simulink model "drone_test-NOAHVUKOSA9F3D"  (R2021b)
settings: Solver=VariableStepAuto  StartTime=0.0  StopTime=10  RelTol=1e-3
values from neighbouring files (symbols this model uses):
  D = [Env.UnrealRiverPts(Env.RiverRegions(i,4),1) Env.UnrealRiverPts(Env.RiverRegions(i,4),2)]    [DefineUAVPath.m]    (also in DistributeIceXML.m; DistributeIceXML1.m; DroneSurveyRegions.m; EstimateIceNumerals.m)
libraries: uavsim3dlib x2, sim3dcameralib x1, sim3dphyssensorlib x1, sim3dlib x1, visionsinks x1
settings Model: Creator=zckog  LastModifiedBy=noahvukosa

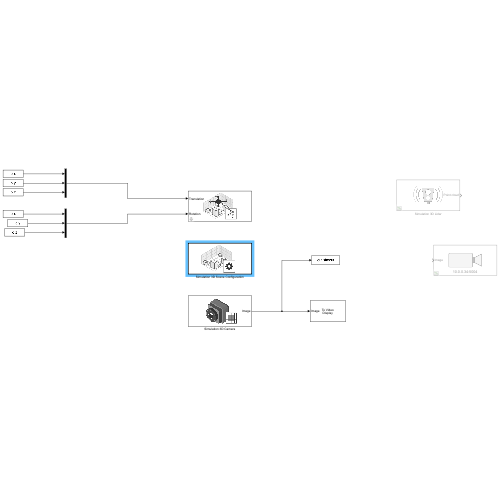
[thumbnail: Simulink's stored preview of the top-level diagram]
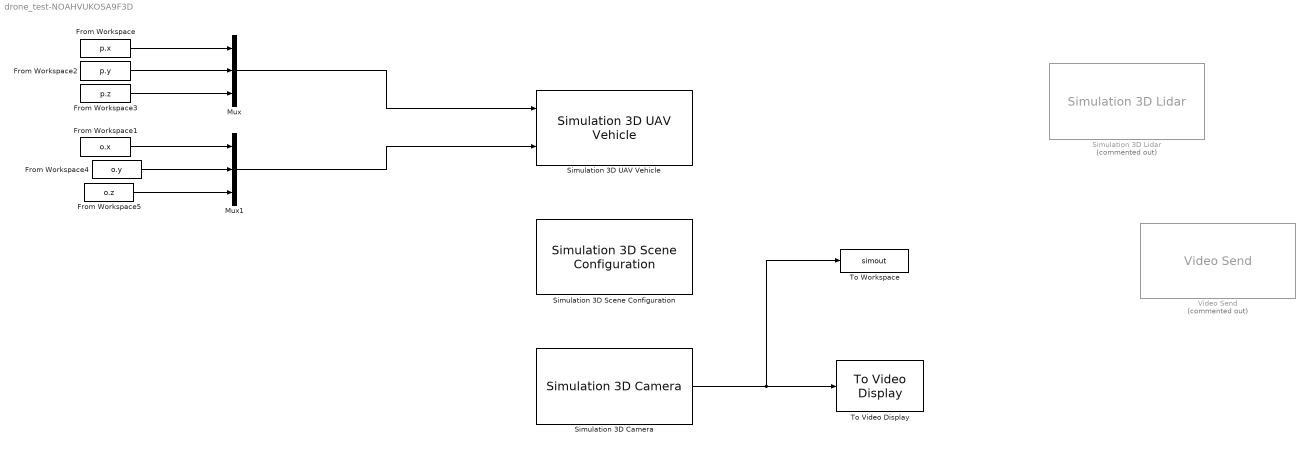
== system drone_test-NOAHVUKOSA9F3D ==
  From Workspace : FromWorkspace  VariableName=p.x
  From Workspace1 : FromWorkspace  VariableName=o.x
  From Workspace2 : FromWorkspace  VariableName=p.y
  From Workspace3 : FromWorkspace  VariableName=p.z
  From Workspace4 : FromWorkspace  VariableName=o.y
  From Workspace5 : FromWorkspace  VariableName=o.z
  Mux : Mux  Inputs=3
  Mux1 : Mux  Inputs=3
  Simulation 3D Camera : sim3dcameralib/Simulation 3D Camera  Priority=1  sensorTag=Sim3dSensor1  sensorId=1  sensorName=Sim3dSensor1  vehTagList={'Scene Origin';'SimulinkVehicle1'}  vehTag=SimulinkVehicle1  mountLoc=Origin  offsetFlag=on  tmountOffset=[0, 0, 0]  extTmount=off  rmountOffset=[0, pi/2, 0]  extRmount=off  FocalLength=[1109, 1109]  OpticalCenter=[640, 360]  ImageSize=[720, 1280]  RadialDistortion=[0, 0]  TangentialDistortion=[0, 0]  SensorSkew=0  DepthOutportEnabled=off  SemanticOutportEnabled=off  TransformOutportEnabled=off  SampleTime=-1  mountPoint=[0 0 0]  mountOrientation=[0 -1.5707963267949 0]  aMode=4  ID=1
      settings: SourceProductBaseCode=AE,DR,UV,VE
  Simulation 3D Lidar : sim3dphyssensorlib/Simulation 3D Lidar  Priority=1  Commented=on  sensorTag=Sim3dSensor2  sensorId=2  sensorName=Sim3dSensor2  vehTagList={'Scene Origin';'SimulinkVehicle1'}  vehTag=SimulinkVehicle1  mountLoc=Origin  offsetFlag=on  tmountOffset=[0, 0, 0]  rmountOffset=[0, 0, 0]  DetectionRange=120  RangeResolution=0.002  VerticalFOV=40  VerticalResolution=1.25  HorizontalFOV=360  HorizontalResolution=0.16  DistanceOutportEnabled=off  TransformOutportEnabled=off  SampleTime=-1  mountPoint=[0 0 0]  mountOrientation=[0 0 0]  aMode=4  ID=2
      settings: SourceProductBaseCode=AE,DR,UV,VE
  Simulation 3D Scene Configuration : sim3dlib/Simulation 3D Scene Configuration  Priority=0  ProjectFormat_internal=Unreal Editor  ProjectFormat=Unreal Editor  SceneDesc=US city block  ProjectName=D:\Matlab2021\toolbox\shared\sim3d_projects\automotive_project\UE4\WindowsNoEditor\VehicleSimulation.exe  ScenePath=/Game/Maps/USCityBlock  UEProjPath=C:\Users\noahvukosa\OneDrive - York University\Documents\DryLandscape\DryLandscape.uproject  vehTagList={'Scene Origin';'SimulinkVehicle1'}  vehTag=SimulinkVehicle1  OpVisEn=off  Ts=1/60  EnableWindow=on  EnableWeather=off  SunAltitude=40.0  SunAzimuth=90  clouds=10  wind=1  fog=0  rain=0  sensorTag=MainCamera1  sensorId=1  sensorName=MainCamera1  mountLoc=Origin  offsetFlag=off  tmountOffset=[0, 0, 0]  rmountOffset=[0, 0, 0]  HorizontalResolution=1280  VerticalResolution=720  HorizontalFOV=60  mountPoint=[0 0 0]  mountOrientation=[0 0 0]  aMode=4  ID=1
      settings: SourceProductBaseCode=AE,DR,UV,VE
  Simulation 3D UAV Vehicle : uavsim3dlib/Simulation 3D UAV Vehicle  Priority=-1  Mesh=Quadrotor  MeshPath=/MathWorksUAVContent/UAVs/HexaRotorUAV/HexaRotor.HexaRotor  Color=Black  ActorName=SimulinkVehicle1  InitialTranslation=[0 0 0]  InitialRotation=[0 0 0]  SampleTime=-1  ActorType=SimulinkVehicle  ID=1  aMode=4  ActorTag=SimulinkVehicle1
      settings: SourceProductBaseCode=UV
  To Video Display : visionsinks/To Video Display  windowSizeMode=Normal  openAtMdlStart=on  fullScreen=off  videoWindowX=536805376  videoWindowY=536805376  saveWindowSize=off  videoWindowWidth=2147483647  videoWindowHeight=2147483647  inputColorFormat=RGB  inputType=Obsolete  imagePorts=One multidimensional signal  OutputDevice=On-screen video monitor  dataOrg=Column-major  isWindowOpen=off
  To Workspace : ToWorkspace  VariableName=simout  SampleTime=-1
  Video Send : uavsim3dlib/Video Send  Commented=on  ImageFormat=RGB  ImageSignal=One multidimensional signal  Compression=JPEG  JPEGQuality=85  VPXFrameDeadline=30  RemoteAddress=10.0.0.34  RemotePort=5004
      settings: SourceProductBaseCode=UV
  wires:
  Mux1/1 -> Simulation 3D UAV Vehicle/2
  Mux/1 -> Simulation 3D UAV Vehicle/1
  From Workspace/1 -> Mux/1
  From Workspace1/1 -> Mux1/1
  From Workspace3/1 -> Mux/3
  From Workspace2/1 -> Mux/2
  From Workspace4/1 -> Mux1/2
  From Workspace5/1 -> Mux1/3
  Simulation 3D Camera/1 -> To Workspace/1, To Video Display/1
